simulink model "SPGF_FSK_0000_R2021b"  (R2021b)
settings: Solver=ode4  StartTime=0.0  StopTime=1.4  FixedStep=50e-6/50  RelTol=1e-3  EnableMultiTasking=on
undefined symbols (not defined in the file): D11, Delta
libraries: spsSeriesRLCBranchLib x1645, spsGroundLib x359, spsCurrentMeasurementLib x145, spsIdealSwitchLib x144, spsStairGeneratorLib x135, spsUniversalBridgeLib x76, spsThreePhaseSeriesRLCLoadLib x57, spsSequenceAnalyzerLib x31, simulink x24, spsThreePhaseParallelRLCLoadLib x20, spsThreePhaseTransformerTwoWindingsLib x20, spsDistributedParametersLineLib x19
(part 31 of 36)

== system SPGF_FSK_0000_R2021b/W60/DPL ==
  Ccs2/1 : spsSeriesRLCBranchLib/Series RLC Branch  LConnTagsString=__new0  RConnTagsString=__new0  BranchType=R  Resistance=-Rg_matrix(3,4)*2  Inductance=1e-3  SetiL0=off  InitialCurrent=0  Capacitance=Rg_matrix(3,4)*2  Setx0=off  InitialVoltage=0  Measurements=None
  Ccs2/3 : spsSeriesRLCBranchLib/Series RLC Branch  LConnTagsString=__new0  RConnTagsString=__new0  BranchType=R  Resistance=-Rg_matrix(3,4)*2  Inductance=1e-3  SetiL0=off  InitialCurrent=0  Capacitance=Rg_matrix(3,4)*2  Setx0=off  InitialVoltage=0  Measurements=None
  Ccs3/1 : spsSeriesRLCBranchLib/Series RLC Branch  LConnTagsString=__new0  RConnTagsString=__new0  BranchType=R  Resistance=-Rg_matrix(5,6)*2  Inductance=1e-3  SetiL0=off  InitialCurrent=0  Capacitance=-C_matrix(5,6)/2  Setx0=off  InitialVoltage=0  Measurements=None
  Ccs3/3 : spsSeriesRLCBranchLib/Series RLC Branch  LConnTagsString=__new0  RConnTagsString=__new0  BranchType=R  Resistance=-Rg_matrix(5,6)*2  Inductance=1e-3  SetiL0=off  InitialCurrent=0  Capacitance=-C_matrix(5,6)/2  Setx0=off  InitialVoltage=0  Measurements=None
  DPL : spsDistributedParametersLineLib/Distributed Parameters Line  Phases=6  Length=LineLength  Frequency=Frequency  Resistance=R_matrix  Inductance=L_matrix  Capacitance=C_matrix  x1=[-0.0001761 -0.638490594647465 0 0 0 -954.812040196447 0;-0.0001758 -0.638604565021584 0 0 0 -954.766295859635 0;-0.0001755 -0.638718529723206 0 0 0 -954.720543041973 0;-0.0001752 -0.638832488751318 0 0 0 -954.674781743869 0;-0.0001749 -0.638946442104909 0 0 0 -954.629011965728 0;-0.0001746 -0.639060389782966 0 0 0 -954.583233707958 0;-0.0001743 -0.639174331784477 0 0 0 -954.537446970965 0;-0.000174 -0.639288268108431 0 0 0 -954.491651755156 0;-0.0001737 -0.639402198753814 0 0 0 -954.445848060937 0;-0.0001734 -0.639516123719615 0 0 0 -954.400035888715 0;-0.0001731 -0.639630043004822 0 0 0 -954.354215238898 0;-0.0001728 -0.639743956608423 0 0 0 -954.308386111892 0;-0.0001725 -0.639857864529406 0 0 0 -954.262548508104 0;-0.0001722 -0.63997176676676 0 0 0 -954.216702427942 0;-0.0001719 -0.640085663319472 0 0 0 -954.170847871813 0;-0.0001716 -0.640199554186532 0 0 0 -954.124984840124 0;-0.0001713 -0.640313439366926 0 0 0 -954.079113333282 0;-0.000171 -0.640427318859645 0 0 0 -954.033233351695 0;-0.0001707 -0.640541192663675 0 0 0 -953.987344895771 0;-0.0001704 -0.640655060778006 0 0 0 -953.941447965917 0;-0.0001701 -0.640768923201627 0 0 0 -953.895542562541 0;-0.0001698 -0.640882779933525 0 0 0 -953.84962868605 0;-0.0001695 -0.640996630972689 0 0 0 -953.803706336852 0;-0.0001692 -0.641110476318109 0 0 0 -953.757775515356 0;-0.0001689 -0.641224315968773 0 0 0 -953.711836221969 0;-0.0001686 -0.641338149923669 0 0 0 -953.665888457099 0;-0.0001683 -0.641451978181787 0 0 0 -953.619932221155 0;-0.000168 -0.641565800742115 0 0 0 -953.573967514544 0;-0.0001677 -0.641679617603643 0 0 0 -953.527994337675 0;-0.0001674 -0.641793428765359 0 0 0 -953.482012690957 0;-0.0001671 -0.641907234226253 0 0 0 -953.436022574798 0;-0.0001668 -0.642021033985313 0 0 0 -953.390023989605 0;-0.0001665 -0.642134828041529 0 0 0 -953.344016935789 0;-0.0001662 -0.64224861639389 0 0 0 -953.298001413757 0;-0.0001659 -0.642362399041385 0 0 0 -953.251977423919 0;-0.0001656 -0.642476175983004 0 0 0 -953.205944966682 0;-0.0001653 -0.642589947217735 0 0 0 -953.159904042457 0;-0.000165 -0.642703712744569 0 0 0 -953.113854651651 0;-0.0001647 -0.642817472562495 0 0 0 -953.067796794674 0;-0.0001644 -0.642931226670502 0 0 0 -953.021730471936 0;-0.0001641 -0.643044975067579 0 0 0 -952.975655683845 0;-0.0001638 -0.643158717752717 0 0 0 -952.92957243081 0;-0.0001635 -0.643272454724906 0 0 0 -952.883480713241 0;-0.0001632 -0.643386185983134 0 0 0 -952.837380531548 0;-0.0001629 -0.643499911526391 0 0 0 -952.791271886139 0;-0.0001626 -0.643613631353668 0 0 0 -952.745154777425 0;-0.0001623 -0.643727345463955 0 0 0 -952.699029205815 0;-0.000162 -0.64384105385624 0 0 0 -952.652895171718 0;-0.0001617 -0.643954756529515 0 0 0 -952.606752675545 0;-0.0001614 -0.644068453482769 0 0 0 -952.560601717705 0;-0.0001611 -0.644182144714992 0 0 0 -952.514442298609 0;-0.0001608 -0.644295830225174 0 0 0 -952.468274418666 0;-0.0001605 -0.644409510012306 0 0 0 -952.422098078287 0;-0.0001602 -0.644523184075378 0 0 0 -952.375913277881 0;-0.0001599 -0.64463685241338 0 0 0 -952.329720017859 0;-0.0001596 -0.644750515025302 0 0 0 -952.283518298631 0;-0.0001593 -0.644864171910135 0 0 0 -952.237308120607 0;-0.000159 -0.644977823066869 0 0 0 -952.191089484199 0;-0.0001587 -0.645091468494494 0 0 0 -952.144862389816 0;-0.0001584 -0.645205108192002 0 0 0 -952.09862683787 0;-0.0001581 -0.645318742158383 0 0 0 -952.05238282877 0;-0.0001578 -0.645432370392627 0 0 0 -952.006130362928 0;-0.0001575 -0.645545992893725 0 0 0 -951.959869440755 0;-0.0001572 -0.645659609660668 0 0 0 -951.913600062661 0;-0.0001569 -0.645773220692446 0 0 0 -951.867322229057 0;-0.0001566 -0.645886825988051 0 0 0 -951.821035940355 0;-0.0001563 -0.646000425546473 0 0 0 -951.774741196965 0;-0.000156 -0.646114019366703 0 0 0 -951.7284379993 0;-0.0001557 -0.646227607447733 0 0 0 -951.682126347769 0;-0.0001554 -0.646341189788552 0 0 0 -951.635806242785 0;-0.0001551 -0.646454766388154 0 0 0 -951.589477684759 0;-0.0001548 -0.646568337245527 0 0 0 ...(+30778 chars)]  x2=[-0.0001761 -0.635125614688809 0 0 0 -961.832428573612 0;-0.0001758 -0.635241691332583 0 0 0 -961.786772243003 0;-0.0001755 -0.635357762333732 0 0 0 -961.741107369184 0;-0.0001752 -0.635473827691223 0 0 0 -961.695433952562 0;-0.0001749 -0.635589887404027 0 0 0 -961.649751993541 0;-0.0001746 -0.635705941471112 0 0 0 -961.604061492528 0;-0.0001743 -0.635821989891447 0 0 0 -961.558362449928 0;-0.000174 -0.635938032664003 0 0 0 -961.512654866148 0;-0.0001737 -0.636054069787746 0 0 0 -961.466938741593 0;-0.0001734 -0.636170101261649 0 0 0 -961.42121407667 0;-0.0001731 -0.636286127084678 0 0 0 -961.375480871784 0;-0.0001728 -0.636402147255805 0 0 0 -961.329739127343 0;-0.0001725 -0.636518161773998 0 0 0 -961.283988843751 0;-0.0001722 -0.636634170638227 0 0 0 -961.238230021416 0;-0.0001719 -0.636750173847461 0 0 0 -961.192462660744 0;-0.0001716 -0.63686617140067 0 0 0 -961.146686762142 0;-0.0001713 -0.636982163296823 0 0 0 -961.100902326016 0;-0.000171 -0.637098149534891 0 0 0 -961.055109352773 0;-0.0001707 -0.637214130113843 0 0 0 -961.009307842819 0;-0.0001704 -0.637330105032648 0 0 0 -960.963497796562 0;-0.0001701 -0.637446074290277 0 0 0 -960.917679214409 0;-0.0001698 -0.6375620378857 0 0 0 -960.871852096765 0;-0.0001695 -0.637677995817886 0 0 0 -960.826016444039 0;-0.0001692 -0.637793948085805 0 0 0 -960.780172256638 0;-0.0001689 -0.637909894688428 0 0 0 -960.734319534969 0;-0.0001686 -0.638025835624724 0 0 0 -960.688458279438 0;-0.0001683 -0.638141770893664 0 0 0 -960.642588490455 0;-0.000168 -0.638257700494218 0 0 0 -960.596710168424 0;-0.0001677 -0.638373624425356 0 0 0 -960.550823313756 0;-0.0001674 -0.638489542686048 0 0 0 -960.504927926857 0;-0.0001671 -0.638605455275265 0 0 0 -960.459024008134 0;-0.0001668 -0.638721362191978 0 0 0 -960.413111557996 0;-0.0001665 -0.638837263435155 0 0 0 -960.367190576849 0;-0.0001662 -0.638953159003769 0 0 0 -960.321261065104 0;-0.0001659 -0.63906904889679 0 0 0 -960.275323023166 0;-0.0001656 -0.639184933113187 0 0 0 -960.229376451445 0;-0.0001653 -0.639300811651932 0 0 0 -960.183421350347 0;-0.000165 -0.639416684511996 0 0 0 -960.137457720283 0;-0.0001647 -0.639532551692349 0 0 0 -960.091485561659 0;-0.0001644 -0.639648413191963 0 0 0 -960.045504874884 0;-0.0001641 -0.639764269009807 0 0 0 -959.999515660367 0;-0.0001638 -0.639880119144853 0 0 0 -959.953517918516 0;-0.0001635 -0.639995963596071 0 0 0 -959.90751164974 0;-0.0001632 -0.640111802362433 0 0 0 -959.861496854447 0;-0.0001629 -0.640227635442911 0 0 0 -959.815473533047 0;-0.0001626 -0.640343462836473 0 0 0 -959.769441685947 0;-0.0001623 -0.640459284542093 0 0 0 -959.723401313556 0;-0.000162 -0.640575100558742 0 0 0 -959.677352416285 0;-0.0001617 -0.640690910885389 0 0 0 -959.631294994541 0;-0.0001614 -0.640806715521008 0 0 0 -959.585229048735 0;-0.0001611 -0.640922514464568 0 0 0 -959.539154579274 0;-0.0001608 -0.641038307715042 0 0 0 -959.493071586568 0;-0.0001605 -0.641154095271401 0 0 0 -959.446980071028 0;-0.0001602 -0.641269877132616 0 0 0 -959.400880033061 0;-0.0001599 -0.64138565329766 0 0 0 -959.354771473078 0;-0.0001596 -0.641501423765503 0 0 0 -959.308654391488 0;-0.0001593 -0.641617188535117 0 0 0 -959.262528788701 0;-0.000159 -0.641732947605474 0 0 0 -959.216394665126 0;-0.0001587 -0.641848700975546 0 0 0 -959.170252021174 0;-0.0001584 -0.641964448644304 0 0 0 -959.124100857254 0;-0.0001581 -0.642080190610721 0 0 0 -959.077941173776 0;-0.0001578 -0.642195926873768 0 0 0 -959.03177297115 0;-0.0001575 -0.642311657432417 0 0 0 -958.985596249786 0;-0.0001572 -0.642427382285641 0 0 0 -958.939411010095 0;-0.0001569 -0.642543101432411 0 0 0 -958.893217252486 0;-0.0001566 -0.642658814871699 0 0 0 -958.84701497737 0;-0.0001563 -0.642774522602478 0 0 0 -958.800804185158 0;-0.000156 -0.642890224623719 0 0 0 -958.75458487626 0;-0.0001557 -0.643005920934396 0 0 0 -958.708357051085 0;-0.0001554 -0.64312161153348 0 0 0 -958.662120710046 0;-0.0001551 -0.643237296419944 0 0 0 -958.615875853553 0;-0.0001548 -0.64335297559276 0 0 0 ...(+30798 chars)]  x3=[-0.0001761 -0.00424604077411073 0 0 0 -385.045035492928 0;-0.0001758 -0.00424830718291609 0 0 0 -385.026974063755 0;-0.0001755 -0.00425057355398525 0 0 0 -385.008909214524 0;-0.0001752 -0.00425283988729808 0 0 0 -384.990840945397 0;-0.0001749 -0.00425510618283445 0 0 0 -384.972769256533 0;-0.0001746 -0.00425737244057423 0 0 0 -384.954694148093 0;-0.0001743 -0.00425963866049728 0 0 0 -384.936615620238 0;-0.000174 -0.00426190484258348 0 0 0 -384.918533673127 0;-0.0001737 -0.00426417098681269 0 0 0 -384.900448306923 0;-0.0001734 -0.00426643709316479 0 0 0 -384.882359521784 0;-0.0001731 -0.00426870316161965 0 0 0 -384.864267317873 0;-0.0001728 -0.00427096919215714 0 0 0 -384.846171695349 0;-0.0001725 -0.00427323518475713 0 0 0 -384.828072654374 0;-0.0001722 -0.0042755011393995 0 0 0 -384.809970195109 0;-0.0001719 -0.00427776705606411 0 0 0 -384.791864317713 0;-0.0001716 -0.00428003293473084 0 0 0 -384.773755022348 0;-0.0001713 -0.00428229877537956 0 0 0 -384.755642309175 0;-0.000171 -0.00428456457799014 0 0 0 -384.737526178354 0;-0.0001707 -0.00428683034254246 0 0 0 -384.719406630047 0;-0.0001704 -0.0042890960690164 0 0 0 -384.701283664415 0;-0.0001701 -0.00429136175739182 0 0 0 -384.683157281618 0;-0.0001698 -0.00429362740764861 0 0 0 -384.665027481817 0;-0.0001695 -0.00429589301976663 0 0 0 -384.646894265174 0;-0.0001692 -0.00429815859372576 0 0 0 -384.62875763185 0;-0.0001689 -0.00430042412950588 0 0 0 -384.610617582005 0;-0.0001686 -0.00430268962708686 0 0 0 -384.592474115801 0;-0.0001683 -0.00430495508644858 0 0 0 -384.574327233399 0;-0.000168 -0.00430722050757092 0 0 0 -384.55617693496 0;-0.0001677 -0.00430948589043376 0 0 0 -384.538023220646 0;-0.0001674 -0.00431175123501696 0 0 0 -384.519866090617 0;-0.0001671 -0.00431401654130041 0 0 0 -384.501705545035 0;-0.0001668 -0.00431628180926399 0 0 0 -384.483541584062 0;-0.0001665 -0.00431854703888758 0 0 0 -384.465374207858 0;-0.0001662 -0.00432081223015105 0 0 0 -384.447203416585 0;-0.0001659 -0.00432307738303428 0 0 0 -384.429029210404 0;-0.0001656 -0.00432534249751716 0 0 0 -384.410851589477 0;-0.0001653 -0.00432760757357956 0 0 0 -384.392670553966 0;-0.000165 -0.00432987261120136 0 0 0 -384.374486104031 0;-0.0001647 -0.00433213761036245 0 0 0 -384.356298239834 0;-0.0001644 -0.0043344025710427 0 0 0 -384.338106961538 0;-0.0001641 -0.00433666749322199 0 0 0 -384.319912269303 0;-0.0001638 -0.00433893237688021 0 0 0 -384.301714163291 0;-0.0001635 -0.00434119722199724 0 0 0 -384.283512643663 0;-0.0001632 -0.00434346202855296 0 0 0 -384.265307710582 0;-0.0001629 -0.00434572679652726 0 0 0 -384.247099364209 0;-0.0001626 -0.00434799152590001 0 0 0 -384.228887604706 0;-0.0001623 -0.0043502562166511 0 0 0 -384.210672432235 0;-0.000162 -0.00435252086876041 0 0 0 -384.192453846956 0;-0.0001617 -0.00435478548220783 0 0 0 -384.174231849033 0;-0.0001614 -0.00435705005697324 0 0 0 -384.156006438628 0;-0.0001611 -0.00435931459303652 0 0 0 -384.137777615901 0;-0.0001608 -0.00436157909037757 0 0 0 -384.119545381015 0;-0.0001605 -0.00436384354897626 0 0 0 -384.101309734132 0;-0.0001602 -0.00436610796881249 0 0 0 -384.083070675413 0;-0.0001599 -0.00436837234986613 0 0 0 -384.064828205022 0;-0.0001596 -0.00437063669211707 0 0 0 -384.046582323119 0;-0.0001593 -0.00437290099554521 0 0 0 -384.028333029868 0;-0.000159 -0.00437516526013042 0 0 0 -384.010080325429 0;-0.0001587 -0.0043774294858526 0 0 0 -383.991824209966 0;-0.0001584 -0.00437969367269163 0 0 0 -383.973564683639 0;-0.0001581 -0.0043819578206274 0 0 0 -383.955301746613 0;-0.0001578 -0.0043842219296398 0 0 0 -383.937035399048 0;-0.0001575 -0.00438648599970871 0 0 0 -383.918765641107 0;-0.0001572 -0.00438875003081404 0 0 0 -383.900492472953 0;-0.0001569 -0.00439101402293566 0 0 0 -383.882215894747 0;-0.0001566 -0.00439327797605346 0 0 0 -383.863935906652 0;-0.0001563 -0.00439554189014734 0 0 0 -383.845652508831 0;-0.000156 -0.00439780576519719 0 0 0 -383.827365701445 0;-0.0001557 -0.00440006960118289 0 0 0 -383.809075484657 0;-0.0001554 ...(+31966 chars)]  x4=[-0.0001761 -0.01784743960928 0 0 0 -376.70962887165 0;-0.0001758 -0.0178494495032123 0 0 0 -376.69145956121 0;-0.0001755 -0.0178514592385944 0 0 0 -376.673286904754 0;-0.0001752 -0.0178534688154082 0 0 0 -376.655110902444 0;-0.0001749 -0.0178554782336361 0 0 0 -376.63693155444 0;-0.0001746 -0.0178574874932601 0 0 0 -376.618748860904 0;-0.0001743 -0.0178594965942624 0 0 0 -376.600562821999 0;-0.000174 -0.0178615055366252 0 0 0 -376.582373437884 0;-0.0001737 -0.0178635143203305 0 0 0 -376.564180708722 0;-0.0001734 -0.0178655229453607 0 0 0 -376.545984634675 0;-0.0001731 -0.0178675314116977 0 0 0 -376.527785215904 0;-0.0001728 -0.0178695397193238 0 0 0 -376.509582452571 0;-0.0001725 -0.0178715478682212 0 0 0 -376.491376344837 0;-0.0001722 -0.017873555858372 0 0 0 -376.473166892864 0;-0.0001719 -0.0178755636897583 0 0 0 -376.454954096814 0;-0.0001716 -0.0178775713623624 0 0 0 -376.436737956849 0;-0.0001713 -0.0178795788761664 0 0 0 -376.418518473131 0;-0.000171 -0.0178815862311524 0 0 0 -376.40029564582 0;-0.0001707 -0.0178835934273027 0 0 0 -376.38206947508 0;-0.0001704 -0.0178856004645994 0 0 0 -376.363839961072 0;-0.0001701 -0.0178876073430246 0 0 0 -376.345607103958 0;-0.0001698 -0.0178896140625606 0 0 0 -376.3273709039 0;-0.0001695 -0.0178916206231896 0 0 0 -376.309131361059 0;-0.0001692 -0.0178936270248936 0 0 0 -376.290888475599 0;-0.0001689 -0.0178956332676549 0 0 0 -376.272642247681 0;-0.0001686 -0.0178976393514557 0 0 0 -376.254392677467 0;-0.0001683 -0.0178996452762782 0 0 0 -376.236139765119 0;-0.000168 -0.0179016510421044 0 0 0 -376.2178835108 0;-0.0001677 -0.0179036566489167 0 0 0 -376.199623914671 0;-0.0001674 -0.0179056620966971 0 0 0 -376.181360976894 0;-0.0001671 -0.017907667385428 0 0 0 -376.163094697633 0;-0.0001668 -0.0179096725150914 0 0 0 -376.144825077048 0;-0.0001665 -0.0179116774856695 0 0 0 -376.126552115303 0;-0.0001662 -0.0179136822971446 0 0 0 -376.10827581256 0;-0.0001659 -0.0179156869494989 0 0 0 -376.089996168981 0;-0.0001656 -0.0179176914427144 0 0 0 -376.071713184729 0;-0.0001653 -0.0179196957767735 0 0 0 -376.053426859965 0;-0.000165 -0.0179216999516583 0 0 0 -376.035137194853 0;-0.0001647 -0.0179237039673511 0 0 0 -376.016844189554 0;-0.0001644 -0.0179257078238339 0 0 0 -375.998547844232 0;-0.0001641 -0.0179277115210891 0 0 0 -375.980248159048 0;-0.0001638 -0.0179297150590988 0 0 0 -375.961945134166 0;-0.0001635 -0.0179317184378452 0 0 0 -375.943638769747 0;-0.0001632 -0.0179337216573106 0 0 0 -375.925329065956 0;-0.0001629 -0.0179357247174771 0 0 0 -375.907016022953 0;-0.0001626 -0.0179377276183269 0 0 0 -375.888699640902 0;-0.0001623 -0.0179397303598423 0 0 0 -375.870379919965 0;-0.000162 -0.0179417329420055 0 0 0 -375.852056860306 0;-0.0001617 -0.0179437353647986 0 0 0 -375.833730462087 0;-0.0001614 -0.0179457376282039 0 0 0 -375.815400725471 0;-0.0001611 -0.0179477397322036 0 0 0 -375.79706765062 0;-0.0001608 -0.0179497416767799 0 0 0 -375.778731237698 0;-0.0001605 -0.0179517434619151 0 0 0 -375.760391486867 0;-0.0001602 -0.0179537450875913 0 0 0 -375.74204839829 0;-0.0001599 -0.0179557465537908 0 0 0 -375.72370197213 0;-0.0001596 -0.0179577478604958 0 0 0 -375.705352208551 0;-0.0001593 -0.0179597490076885 0 0 0 -375.686999107715 0;-0.000159 -0.0179617499953512 0 0 0 -375.668642669785 0;-0.0001587 -0.017963750823466 0 0 0 -375.650282894924 0;-0.0001584 -0.0179657514920152 0 0 0 -375.631919783295 0;-0.0001581 -0.0179677520009811 0 0 0 -375.613553335062 0;-0.0001578 -0.0179697523503458 0 0 0 -375.595183550387 0;-0.0001575 -0.0179717525400916 0 0 0 -375.576810429434 0;-0.0001572 -0.0179737525702007 0 0 0 -375.558433972366 0;-0.0001569 -0.0179757524406554 0 0 0 -375.540054179346 0;-0.0001566 -0.0179777521514378 0 0 0 -375.521671050537 0;-0.0001563 -0.0179797517025303 0 0 0 -375.503284586103 0;-0.000156 -0.0179817510939151 0 0 0 -375.484894786207 0;-0.0001557 -0.0179837503255744 0 0 0 -375.466501651013 0;-0.0001554 -0.0179857493974904 0 0 0 -375.448105180683 0;-0.0001551 -0.0179877483096454 0 ...(+31368 chars)]  x5=0.000175937547208628  V1=ones(3,3)  V2=ones(3,3)  I1=ones(3,3)  I2=ones(3,3)  nHarmo=1  Measurements=None  Decoupling=off  VsMag0=0  VrMag0=0  VsAngle0=0  VrAngle0=0  IsMag0=0  IrMag0=0  IsAngle0=0  IrAngle0=0
  Ground{1..4} (4 alike) : spsGroundLib/Ground  LConnTagsString=a
  Rcs*1 : spsSeriesRLCBranchLib/Series RLC Branch  LConnTagsString=__new0  RConnTagsString=__new0  BranchType=R  Resistance=-Rg_matrix(1,2)*2  Inductance=1e-3  SetiL0=off  InitialCurrent=0  Capacitance=Rg_matrix(1,2)*2  Setx0=off  InitialVoltage=0  Measurements=None
  Rcs*2 : spsSeriesRLCBranchLib/Series RLC Branch  LConnTagsString=__new0  RConnTagsString=__new0  BranchType=R  Resistance=-Rg_matrix(1,2)*2  Inductance=1e-3  SetiL0=off  InitialCurrent=0  Capacitance=Rg_matrix(1,2)*2  Setx0=off  InitialVoltage=0  Measurements=None
  Rgsg1/1 : spsSeriesRLCBranchLib/Series RLC Branch  LConnTagsString=__new0  RConnTagsString=__new0  BranchType=R  Resistance=(Rg_matrix(4,4)+Rg_matrix(3,4))*2  Inductance=1e-3  SetiL0=off  InitialCurrent=0  Capacitance=Rg_matrix(1,2)*2  Setx0=off  InitialVoltage=0  Measurements=None
  Rgsg1/2 : spsSeriesRLCBranchLib/Series RLC Branch  LConnTagsString=__new0  RConnTagsString=__new0  BranchType=R  Resistance=(Rg_matrix(2,2)+Rg_matrix(1,2))*2  Inductance=1e-3  SetiL0=off  InitialCurrent=0  Capacitance=Rg_matrix(1,2)*2  Setx0=off  InitialVoltage=0  Measurements=None
  Rgsg1/3 : spsSeriesRLCBranchLib/Series RLC Branch  LConnTagsString=__new0  RConnTagsString=__new0  BranchType=R  Resistance=(Rg_matrix(4,4)+Rg_matrix(3,4))*2  Inductance=1e-3  SetiL0=off  InitialCurrent=0  Capacitance=Rg_matrix(1,2)*2  Setx0=off  InitialVoltage=0  Measurements=None
  Rgsg1/4 : spsSeriesRLCBranchLib/Series RLC Branch  LConnTagsString=__new0  RConnTagsString=__new0  BranchType=R  Resistance=(Rg_matrix(2,2)+Rg_matrix(1,2))*2  Inductance=1e-3  SetiL0=off  InitialCurrent=0  Capacitance=Rg_matrix(1,2)*2  Setx0=off  InitialVoltage=0  Measurements=None
  Rsg*1 : spsSeriesRLCBranchLib/Series RLC Branch  LConnTagsString=__new0  RConnTagsString=__new0  BranchType=R  Resistance=(Rg_matrix(6,6)+Rg_matrix(5,6))*2  Inductance=1e-3  SetiL0=off  InitialCurrent=0  Capacitance=Rg_matrix(1,2)*2  Setx0=off  InitialVoltage=0  Measurements=None
  Rsg*2 : spsSeriesRLCBranchLib/Series RLC Branch  LConnTagsString=__new0  RConnTagsString=__new0  BranchType=R  Resistance=(Rg_matrix(6,6)+Rg_matrix(5,6))*2  Inductance=1e-3  SetiL0=off  InitialCurrent=0  Capacitance=Rg_matrix(1,2)*2  Setx0=off  InitialVoltage=0  Measurements=None
  A : PMIOPort  Side=Left
  B : PMIOPort  Port=2  Side=Left
  C : PMIOPort  Port=3  Side=Left
  a : PMIOPort  Port=4  Side=Right
  b : PMIOPort  Port=5  Side=Right
  c : PMIOPort  Port=6  Side=Right
  connections:
  A/RConn1 -- DPL/LConn1 -- Rcs*2/RConn1
  B/RConn1 -- DPL/LConn3 -- Ccs2/3/RConn1
  C/RConn1 -- DPL/LConn5 -- Ccs3/3/RConn1
  Rgsg1/2/RConn1 -- Rsg*2/RConn1 -- Rgsg1/1/RConn1 -- Ground2/LConn1
  DPL/LConn2 -- Rcs*2/LConn1 -- Rgsg1/2/LConn1 -- DPL/LConn4 -- Ccs2/3/LConn1 -- Rgsg1/1/LConn1 -- DPL/LConn6 -- Rsg*2/LConn1 -- Ccs3/3/LConn1 -- Ground3/LConn1
  Rgsg1/3/RConn1 -- Rsg*1/RConn1 -- Rgsg1/4/RConn1 -- Ground1/LConn1
  Rgsg1/3/LConn1 -- Ccs2/1/LConn1 -- DPL/RConn4 -- DPL/RConn2 -- Rgsg1/4/LConn1 -- Rcs*1/LConn1 -- Rsg*1/LConn1 -- Ccs3/1/LConn1 -- DPL/RConn6 -- Ground4/LConn1
  Rcs*1/RConn1 -- DPL/RConn1 -- a/RConn1
  DPL/RConn3 -- Ccs2/1/RConn1 -- b/RConn1
  DPL/RConn5 -- Ccs3/1/RConn1 -- c/RConn1
